simulink subsystem "Final_Project_PreAlign_20260605_152612"  (R2024a)
settings: Solver=VariableStepAuto  StartTime=0.0  StopTime=10.0  RelTol=1e-3
values from neighbouring files (symbols this model uses):
  D = hypot(Ep(:,1)-Tp(:,1)',Ep(:,2)-Tp(:,2)')    [pp_compare_stage.m]    (also in pp_diag_path.m; pp_t09_clear.m = hypot(Ep(:,1)-Tperim(:,1)', Ep(:,2)-Tperim(:,2)'); pp_tune2.m)
undefined symbols (not defined in the file or in its folder): waypoint_const
libraries: CarMaker4SL x83, simulink x2
(part 4 of 5)

== matlab function Final_Project_PreAlign_20260605_152612/Driving_Module_Ver.3_PSH/Subsystem/Controller ==
  data: ego_cross_track_err input; steer output; ego_head_err input; ego_max_curvature input; target_speed input; lead_dist input; lead_speed input; drive_state input; lane_settled input; submission_state input; ego_state input; accel output; front_dist_lock output; gear_pos output double
function [steer, accel, front_dist_lock, gear_pos] = controller(...
    ego_cross_track_err, ego_head_err, ego_max_curvature, target_speed, ...
    lead_dist, lead_speed, drive_state, lane_settled, submission_state, ego_state)
%#codegen

    % ============================================================
    % 기본 상수
    % ============================================================
    TS           = 0.01;
    STEER_LIM    = 0.58;
    MAX_SPEED    = 50.0;
    MODE_LCHG    = int32(1);
    MODE_PARK    = int32(2);
    KAPPA_EPS    = 1e-4;
    SPD_DEADBAND = 0.3;

    % ============================================================
    % Cmd 정의
    % 0 : 일반 주행
    % 1 : 주차장 진입
    % 2 : 톨게이트
    % ============================================================
    CMD_DRIVE = int32(0); %#ok<NASGU>
    CMD_PARK  = int32(1);
    CMD_TOLL  = int32(2);

    submission_i = int32(round(double(submission_state)));

    mandatory_follow = (submission_i == CMD_PARK) || (submission_i == CMD_TOLL);

    % ============================================================
    % Ego unpack
    % ============================================================
    ego_x = ego_state.Car_Fr1_tx;
    ego_y = ego_state.Car_Fr1_ty;
    ego_v = ego_state.Ego_V;

    if ego_v > 60.0
        ego_v = ego_v / 3.6;
    end

    if ego_v < 0.0
        ego_v = 0.0;
    end

    % ============================================================
    % Parking waypoints
    % ============================================================
    L4_X     = -46.856;  L4_Y     = 15.842;
    L5_END_X =  2.617;   L5_END_Y = -35.0;

    dist_l4     = sqrt((ego_x - L4_X)^2     + (ego_y - L4_Y)^2);
    dist_to_end = sqrt((ego_x - L5_END_X)^2 + (ego_y - L5_END_Y)^2);

    % ============================================================
    % 파라미터 정의: 일반 주행 / 주차 진입
    % ============================================================
    K_STANLEY_NRM  = 0.88;   K_STANLEY_PRK  = 0.45;
    KP_HEAD_NRM    = 0.90;   KP_HEAD_PRK    = 0.50;
    LOOK_FRONT_NRM = calcLookFront(ego_v);  LOOK_FRONT_PRK = 10.0;
    ALAT_NRM       = 3.50;   ALAT_PRK       = 1.50;
    ATOT_NRM       = 4.00;   ATOT_PRK       = 2.00;
    MCSPD_NRM      = 7.00;   MCSPD_PRK      = 1.00;
    VREF_A_NRM     = 50.0;   VREF_A_PRK     = 2.00;
    VREF_D_NRM     = 100.0;  VREF_D_PRK     = 5.00;
    JERK_U_NRM     = 50.0;   JERK_U_PRK     = 3.00;
    JERK_D_NRM     = 60.0;   JERK_D_PRK     = 5.00;
    AMAX_NRM       = 10.0;   AMAX_PRK       = 3.00;
    DMAX_NRM       = 10.0;   DMAX_PRK       = 5.00;

    FADE_FAR  = 50.0;
    FADE_NEAR = 20.0;

    if submission_i == CMD_PARK
        if dist_l4 >= FADE_FAR
            r = 0.0;
        elseif dist_l4 <= FADE_NEAR
            r = 1.0;
        else
            r = (FADE_FAR - dist_l4) / (FADE_FAR - FADE_NEAR);
        end
    else
        r = 0.0;
    end

    K_STANLEY       = K_STANLEY_NRM  + r * (K_STANLEY_PRK  - K_STANLEY_NRM);
    KP_HEAD         = KP_HEAD_NRM    + r * (KP_HEAD_PRK    - KP_HEAD_NRM);
    LOOK_FRONT      = LOOK_FRONT_NRM + r * (LOOK_FRONT_PRK - LOOK_FRONT_NRM);
    A_LAT_LIMIT     = ALAT_NRM       + r * (ALAT_PRK       - ALAT_NRM);
    A_TOTAL_LIMIT   = ATOT_NRM       + r * (ATOT_PRK       - ATOT_NRM);
    MIN_CURVE_SPEED = MCSPD_NRM      + r * (MCSPD_PRK      - MCSPD_NRM);
    V_REF_ACCEL     = VREF_A_NRM     + r * (VREF_A_PRK     - VREF_A_NRM);
    V_REF_DECEL     = VREF_D_NRM     + r * (VREF_D_PRK     - VREF_D_NRM);
    JERK_UP         = JERK_U_NRM     + r * (JERK_U_PRK     - JERK_U_NRM);
    JERK_DOWN       = JERK_D_NRM     + r * (JERK_D_PRK     - JERK_D_NRM);
    ACCEL_MAX_BASE  = AMAX_NRM       + r * (AMAX_PRK       - AMAX_NRM);
    DECEL_MAX_BASE  = DMAX_NRM       + r * (DMAX_PRK       - DMAX_NRM);

    % ============================================================
    % L4 통과 latch
    % ============================================================
    persistent l4_passed_p l4_pass_init_p

    if isempty(l4_pass_init_p)
        l4_passed_p    = false;
        l4_pass_init_p = true;
    end

    if submission_i ~= CMD_PARK
        l4_passed_p = false;
    end

    L4_PASS_DIST = 3.0;

    if submission_i == CMD_PARK && dist_l4 < L4_PASS_DIST
        l4_passed_p = true;
    end

    % ============================================================
    % 목표속도 결정
    % ============================================================
    if submission_i == CMD_PARK

        DECEL_DIST = 25.0;
        STOP_DIST  =  2.0;

        SPD_BEFORE_L4_FAR  = 12.3;
        SPD_BEFORE_L4_NEAR = 4.8;
        SPD_AFTER_L4       = 5.8;
        SPD_PARK_INSIDE    = 4.2;

        if drive_state == MODE_PARK

            if dist_to_end < STOP_DIST
                ts = 0.0;
            elseif dist_to_end < DECEL_DIST
                ts = SPD_PARK_INSIDE * (dist_to_end / DECEL_DIST);
            else
                ts = SPD_PARK_INSIDE;
            end

        elseif l4_passed_p

            ts = SPD_AFTER_L4;

        elseif dist_l4 > FADE_NEAR

            if dist_l4 >= FADE_FAR
                ts = SPD_BEFORE_L4_FAR;
            else
                ts = SPD_BEFORE_L4_FAR + ...
                     (SPD_BEFORE_L4_NEAR - SPD_BEFORE_L4_FAR) * r;
            end

        else

            ts = SPD_AFTER_L4;

        end

    else

        ts = target_speed;

        if ts > 20.0
            ts = ts / 3.6;
        end

    end

    if ts > MAX_SPEED
        ts = MAX_SPEED;
    end

    if ts < 0.0
        ts = 0.0;
    end

    % ============================================================
    % persistent
    % ============================================================
    persistent desired_v_p accel_p did_init

    if isempty(did_init)
        desired_v_p = ego_v;
        accel_p     = 0.0;
        did_init    = true;
    end

    % ============================================================
    % 1. Stanley 조향
    % ============================================================
    v_safe = ego_v;

    if v_safe < 1.0
        v_safe = 1.0;
    end

    steer = KP_HEAD * ego_head_err - atan2(K_STANLEY * ego_cross_track_err, v_safe);

    if steer > STEER_LIM
        steer = STEER_LIM;
    elseif steer < -STEER_LIM
        steer = -STEER_LIM;
    end

    % ============================================================
    % 1-1. 끝점 추가 좌회전 블렌드
    % ============================================================
    EXTRA_DIST = 5.0;
    EXTRA_RAD  = pi / 3.0;

    if submission_i == CMD_PARK && drive_state == MODE_PARK
        if dist_to_end < EXTRA_DIST && dist_to_end > 0.0
            blend = 1.0 - (dist_to_end / EXTRA_DIST);
            steer = steer + blend * EXTRA_RAD;

            if steer > EXTRA_RAD
                steer = EXTRA_RAD;
            elseif steer < -EXTRA_RAD
                steer = -EXTRA_RAD;
            end
        end
    end

    % ============================================================
    % 2. 곡률 기반 목표속도 제한
    % ============================================================
    desired_v_raw = ts;

    if ego_max_curvature > KAPPA_EPS

        v_curve = sqrt(A_LAT_LIMIT / ego_max_curvature);

        if v_curve < MIN_CURVE_SPEED
            v_curve = MIN_CURVE_SPEED;
        end

        if v_curve < desired_v_raw
            desired_v_raw = v_curve;
        end
    end

    % ============================================================
    % 3. ACC 앞차 감속
    % ============================================================
    acc_active = false;

    if mandatory_follow

        LOOK_FRONT_ACC = LOOK_FRONT;

        if LOOK_FRONT_ACC < 45.0
            LOOK_FRONT_ACC = 45.0;
        end

        if lead_dist < LOOK_FRONT_ACC
            acc_active = true;
        end

    else

        if drive_state ~= MODE_PARK

            if lead_dist < LOOK_FRONT

                time_gap = 2.0;
                ACC_GAIN = 0.5;

                safe_v = lead_speed + (lead_dist - time_gap * ego_v) * ACC_GAIN;

                if safe_v < desired_v_raw
                    desired_v_raw = safe_v;
                end
            end
        end
    end

    if desired_v_raw < 0.0
        desired_v_raw = 0.0;
    end

    % ============================================================
    % 4. 목표속도 변화율 제한
    % ============================================================
    dv = desired_v_raw - desired_v_p;

    max_dv_up = V_REF_ACCEL * TS;
    max_dv_dn = V_REF_DECEL * TS;

    if dv > max_dv_up
        desired_v_p = desired_v_p + max_dv_up;
    elseif dv < -max_dv_dn
        desired_v_p = desired_v_p - max_dv_dn;
    else
        desired_v_p = desired_v_raw;
    end

    desired_v = desired_v_p;

    if mandatory_follow && acc_active
        desired_v_p = ego_v;
        desired_v   = ego_v;
    end

    % ============================================================
    % 5. 가감속
    % ============================================================
    spd_err = desired_v - ego_v;

    if mandatory_follow && acc_active

        lead_v = lead_speed;

        if lead_v > 60.0
            lead_v = lead_v / 3.6;
        end

        if lead_v < 0.0
            lead_v = 0.0;
        end

        TIME_GAP_MAND     = 2.0;
        STOP_BUFFER       = 6.0;
        LOW_SPEED_MIN_GAP = 10.0;

        safe_gap = STOP_BUFFER + TIME_GAP_MAND * ego_v;

        if ego_v < 6.0
            if safe_gap < LOW_SPEED_MIN_GAP
                safe_gap = LOW_SPEED_MIN_GAP;
            end
        end

        gap_err   = lead_dist - safe_gap;
        closing_v = ego_v - lead_v;

        if closing_v < 0.0
            closing_v = 0.0;
        end

        GAP_CLOSE = -1.5;
        GAP_FAR   =  4.0;

        ACC_FOLLOW_ACCEL_MAX = 0.35;
        ACC_MATCH_ACCEL_MAX  = 0.20;
        ACC_FOLLOW_DECEL_MAX = 5.5;

        KP_FAR   = 0.05;
        KP_MATCH = 0.60;
        KP_CLOSE = 0.35;
        KD_CLOSE = 1.40;

        if gap_err > GAP_FAR

            accel_cmd = KP_FAR * (gap_err - GAP_FAR);

            if accel_cmd > ACC_FOLLOW_ACCEL_MAX
                accel_cmd = ACC_FOLLOW_ACCEL_MAX;
            end

            MAX_CATCHUP_V = 0.5;

            if ego_v > lead_v + MAX_CATCHUP_V
                accel_cmd = 0.0;
            end

        elseif gap_err < GAP_CLOSE

            accel_cmd = KP_CLOSE * gap_err - KD_CLOSE * closing_v;

            if accel_cmd < -ACC_FOLLOW_DECEL_MAX
                accel_cmd = -ACC_FOLLOW_DECEL_MAX;
            end

        else

            accel_cmd = KP_MATCH * (lead_v - ego_v);

            if accel_cmd > ACC_MATCH_ACCEL_MAX
                accel_cmd = ACC_MATCH_ACCEL_MAX;
            elseif accel_cmd < -ACC_FOLLOW_DECEL_MAX
                accel_cmd = -ACC_FOLLOW_DECEL_MAX;
            end
        end

        if lead_v < 0.3 && lead_dist < safe_gap + 5.0
            if accel_cmd > 0.0
                accel_cmd = 0.0;
            end
        end

        % 비상감속 조건 완화
        EMERGENCY_GAP = 5.0 + 0.5 * ego_v;

        if ego_v < 6.0
            EMERGENCY_GAP = 7.0 + 0.5 * ego_v;
        end

        if lead_dist < EMERGENCY_GAP && closing_v > 1.0
            accel_cmd = -ACC_FOLLOW_DECEL_MAX;
        end

    elseif submission_i == CMD_PARK

        KP_SPD = 2.0;
        accel_cmd = KP_SPD * spd_err;

        if accel_cmd > ACCEL_MAX_BASE
            accel_cmd = ACCEL_MAX_BASE;
        elseif accel_cmd < -DECEL_MAX_BASE
            accel_cmd = -DECEL_MAX_BASE;
        end

    else

        if spd_err > SPD_DEADBAND
            accel_cmd = ACCEL_MAX_BASE;
        elseif spd_err < -SPD_DEADBAND
            accel_cmd = -DECEL_MAX_BASE;
        else
            accel_cmd = 0.5 * spd_err;
        end
    end

    % ============================================================
    % 6. Friction circle 기반 가속 한계
    % ============================================================
    a_lat_now = ego_v * ego_v * ego_max_curvature;

    if a_lat_now >= A_TOTAL_LIMIT
        a_lon_avail = 0.5;
    else
        a_lon_avail = sqrt(A_TOTAL_LIMIT * A_TOTAL_LIMIT - a_lat_now * a_lat_now);

        if a_lon_avail < 0.5
            a_lon_avail = 0.5;
        end
    end

    accel_max = ACCEL_MAX_BASE;

    if a_lon_avail < accel_max
        accel_max = a_lon_avail;
    end

    if accel_cmd > accel_max
        accel_cmd = accel_max;
    end

    if accel_cmd < -DECEL_MAX_BASE
        accel_cmd = -DECEL_MAX_BASE;
    end

    % ============================================================
    % 7. Jerk 제한
    % ============================================================
    da = accel_cmd - accel_p;

    if mandatory_follow && acc_active

        FOLLOW_JERK_UP      = 0.8;
        FOLLOW_JERK_RELEASE = 4.0;
        FOLLOW_JERK_DOWN    = 80.0;

        if accel_p < 0.0
            max_da_up = FOLLOW_JERK_RELEASE * TS;
        else
            max_da_up = FOLLOW_JERK_UP * TS;
        end

        max_da_dn = FOLLOW_JERK_DOWN * TS;

    else

        max_da_up = JERK_UP   * TS;
        max_da_dn = JERK_DOWN * TS;
    end

    if da > max_da_up
        accel_p = accel_p + max_da_up;
    elseif da < -max_da_dn
        accel_p = accel_p - max_da_dn;
    else
        accel_p = accel_cmd;
    end

    accel = accel_p;

    % ============================================================
    % 8. front_dist_lock
    % ============================================================
    if drive_state == MODE_LCHG || lane_settled
        front_dist_lock = 0;
    else
        front_dist_lock = lead_dist;
    end

    % ============================================================
    % 9. Gear Position
    % ============================================================
    gear_pos = double(1);

end


function LOOK_FRONT = calcLookFront(v)
%#codegen

    v = abs(v);

    if v > 60.0
        v = v / 3.6;
    end

    V_HIGH = 80.0 / 3.6;

    if v < V_HIGH
        LOOK_FRONT = 25.0 + 1.0 * v;
    else
        LOOK_FRONT = 50.0 + 1.0 * V_HIGH + 30.0 * (v - V_HIGH);
    end

    if LOOK_FRONT > 120.0
        LOOK_FRONT = 120.0;
    end

end

== matlab function Final_Project_PreAlign_20260605_152612/Module_Selector/parking_entry_selector ==
  data: parking_map input; module_select output; parking_goal input; parking_start input; ego_global_pos input; waypoints input
function module_select = parking_entry_selector(parking_map, parking_goal, parking_start, ego_global_pos, waypoints) %#codegen
% Module_Selector 상태 (출력 module_select):
%   0 = Driving, 1 = Parking(도달 시 래치 고정), 2 = Tollgate(구간), 3 = 주차목표 도달(래치 고정)
%   톨게이트: (-94.9269,-159.103) 도달 -> 2,  (-172.724,-86.2036) 통과 -> 0
%   주차    : (-141.562,-17.5155) 도달 -> 1 로 래치
%   주차목표: (-2.92924, 9.6997) 도달 -> 3 으로 래치 (최우선)
%   ego_global_pos = [x; y] (Bus Selector+Mux)

persistent parking_latched tollgate_active goal_latched
if isempty(parking_latched)
    parking_latched = false;
end
if isempty(tollgate_active)
    tollgate_active = false;
end
if isempty(goal_latched)
    goal_latched = false;
end

TG_START = [-94.9269, -159.103];   % 톨게이트 시작
TG_END   = [-172.724,  -86.2036];  % 톨게이트 끝
PARK_REF = [-141.562,  -17.5155];  % 주차 진입
GOAL_REF = [1.81923,    -36.6415];  % 주차 목표 지점 (state 3)
R = 6.0;                           % 도달 인정 반경 [m] (자차가 ~5m 옆으로 지나가서 키움)
R_GOAL = 3.0;                      % 주차 목표 도달 반경 [m] (진입로 라인과 구분되도록 작게)

ex = ego_global_pos(1);
ey = ego_global_pos(2);

if hypot(ex - TG_START(1), ey - TG_START(2)) <= R
    tollgate_active = true;
end
if hypot(ex - TG_END(1), ey - TG_END(2)) <= R
    tollgate_active = false;
end

if hypot(ex - PARK_REF(1), ey - PARK_REF(2)) <= R
    parking_latched = true;
end

if hypot(ex - GOAL_REF(1), ey - GOAL_REF(2)) <= R_GOAL
    goal_latched = true;
end

if goal_latched
    module_select = 3.0;
elseif parking_latched
    module_select = 1.0;
elseif tollgate_active
    module_select = 2.0;
else
    module_select = 0.0;
end
end

== stateflow chart Final_Project_PreAlign_20260605_152612/FcnRouter_State ==
  (default) -> (junction 5)
  (junction 5) -> (junction 7) [order 1] : [isPark]{call_park;}
  (junction 5) -> (junction 8) [order 2] : [isPark == 0]{call_drive;}
  data: isPark input double
  events: tick input FUNCTION_CALL_EVENT; call_drive output FUNCTION_CALL_EVENT; call_park output FUNCTION_CALL_EVENT

== matlab function Final_Project_PreAlign_20260605_152612/Parking_system/MATLAB Function2 ==
  settings: sampleTime=0.05
  data: map_boundary input; mapMatrix output size=[200 200]; traffic_info input; traffic_size input
function mapMatrix = generate_map_(map_boundary, traffic_info, traffic_size)
%GENERATE_MAP_  Self-contained version of the "MATLAB Function1" block.
%   Source model : Models/Day4_5/Day4_5_Scenario_1.slx
%   Block path   : CarMaker/Subsystem/Day4 & 5/Scenario 1/MATLAB Function1
%
%   The block body only calls the pp_* helper; this file additionally
%   bundles every pp_*.m it transitively depends on as local functions,
%   so it runs standalone without dev/day4_5/pp_*.m on the MATLAB path.
%
%   Bundled dependencies (5): pp_generate_map, pp_cfg, pp_entrance_path, pp_grid2world, pp_world2grid
mapMatrix = pp_generate_map(map_boundary, traffic_info, traffic_size);
end

% ========================================================================
%  Local dependency functions (bundled verbatim from dev/day4_5/pp_*.m).
%  Do not edit here; edit the pp_*.m sources and re-bundle.
% ========================================================================

function mapMatrix = pp_generate_map(map_boundary, traffic_info, traffic_size) %#ok<INUSD>
%#codegen
% PP_GENERATE_MAP  Base occupancy grid for the parking area (M2 logic).
%   Output mapMatrix is n-by-n, indexed (iy, ix): 0 = free, 1 = occupied.
%
%   Drivable space = the parking-lot rectangle (cfg.lot) UNION the entrance-road
%   corridor (route5 centerline +- halfw, from pp_entrance_path), each inset by
%   cfg.edge_margin. Everything else inside cfg.bounds is OCCUPIED, so the planner
%   cannot cut across non-road area. Static parked cars are stamped afterwards by
%   pp_add_obstacle.
%
%   PERFORMANCE: the map is STATIC, so it is computed ONCE and cached in a
%   persistent (this block runs every sim step; the corridor distance-carve must
%   not run per-step). Codegen rule: the persistent is assigned inside the
%   `if isempty(...)` guard BEFORE it is read. Cache clears at sim start and by
%   `clear functions` after editing cfg / pp_entrance_path.
%
%   map_boundary / traffic_info / traffic_size are accepted only for MATLAB
%   Function block signature compatibility (intentionally unused here).
persistent BASE
if isempty(BASE)
    cfg = pp_cfg();
    n = cfg.n; b = cfg.bounds; em = cfg.edge_margin;
    M = ones(n, n);                                 % default OCCUPIED; carve drivable area free

    % --- carve the REAL drivable surface FREE (IPGRoad geometry, not a rectangle) -
    %   Driving lanes (type 0) + parking bay (type 13), reconstructed from the
    %   TestRun road links/lanes. surf rows = [x0 x1 y0 y1], ALREADY inset by the
    %   edge margin on OUTER paved walls only; internal seams (Vroad<->Hstrip and
    %   Hstrip<->Bay) are left flush so the vehicle can cross between them.
    %   Everything else inside cfg.bounds stays OCCUPIED (no cutting across void).
    %     Vroad : x~0 vertical driving road     world x[-2.5,2.5] y[-36.6,6]
    %     Hstrip: y~-36.6 driving strip (type0)  world x[0,47.6]   y[-39.1,-34.1]
    %     Bay   : type-13 parking bay (north)    world x[5.5,47.6] y[-34.1,-4.1]
    %     BayW  : narrow west sliver of the bay  world x[4,5.5]    y[-34.1,-30.1]
    surf = [ -2.3  2.3  -36.6    6.0 ;
              0.0 47.4  -38.9  -34.1 ;
              5.7 47.4  -34.1   -4.3 ;
              4.0  5.5  -34.1  -30.1 ];
    for r = 1:size(surf,1)
        [sx0, sy0] = pp_world2grid(surf(r,1), surf(r,3), b, n);
        [sx1, sy1] = pp_world2grid(surf(r,2), surf(r,4), b, n);
        for ix = min(sx0,sx1):max(sx0,sx1)
            for iy = min(sy0,sy1):max(sy0,sy1)
                M(iy, ix) = 0;
            end
        end
    end

    % --- occupied border ring (keeps the search bounded) ----------------------
    w = cfg.wall_cells;
    if w > 0
        M(1:w, :)     = 1;
        M(n-w+1:n, :) = 1;
        M(:, 1:w)     = 1;
        M(:, n-w+1:n) = 1;
    end

    BASE = M;
end
mapMatrix = BASE;
end

% ===== distance from point (px,py) to segment (ax,ay)-(bx,by) ==============
function d = seg_dist_(px, py, ax, ay, bx, by)
%#codegen
vx = bx-ax; vy = by-ay;
wx = px-ax; wy = py-ay;
vv = vx*vx + vy*vy;
if vv < 1e-9
    d = hypot(px-ax, py-ay); return;
end
t = (wx*vx + wy*vy) / vv;
if t < 0, t = 0; elseif t > 1, t = 1; end
qx = ax + t*vx; qy = ay + t*vy;
d = hypot(px-qx, py-qy);
end

function cfg = pp_cfg()
%#codegen
% PP_CFG  Configuration for the Day4/5 precise-parking controller (Kia_EV6).
%   Geometry from Data/Vehicle/Kia_EV6 (Vehicle.OuterSkin & wheel positions).
%
%   Pose convention (CarMaker): Car.Fr1 origin = REAR-BUMPER center on the road,
%   X forward, Y left, yaw = Car.Fr1.rz [rad]. Same convention for the mission
%   goal pose and every obstacle coordinate. Internal planning/tracking uses the
%   REAR AXLE, d_r ahead of Fr1:  rear_axle = Fr1 + d_r*[cos(yaw) sin(yaw)].
%
%   CODEGEN NOTE: build every struct field from LOCAL variables / literals only.
%   Never read a cfg field while still constructing cfg.

% --- local geometry constants (Kia_EV6) -----------------------------------
veh_L     = 4.68;
veh_W     = 1.88;
wheelbase = 2.90;
d_r       = 0.95;
delta_max = 30*pi/180;

% --- vehicle ---------------------------------------------------------------
cfg.veh_L       = veh_L;
cfg.veh_W       = veh_W;
cfg.veh_halfW   = veh_W/2;
cfg.wheelbase   = wheelbase;
cfg.track_f     = 1.624;                  % front track width [m] (wheels at y=+-0.812)
cfg.d_r         = d_r;
cfg.foot_ahead  = veh_L - d_r;            % rear-axle -> front bumper [m] = 3.73
cfg.foot_behind = d_r;                    % rear-axle -> rear bumper  [m] = 0.95
cfg.delta_max   = delta_max;
cfg.Rmin        = wheelbase / tan(delta_max);

% --- obstacle vehicle (IPG_CompanyCar_2018_Blue) ---------------------------
cfg.obs_L       = 4.47;
cfg.obs_W       = 1.97;
cfg.holdout     = 0;                     % pp_obstacles row kept FREE as the parking
                                          %   target (held-out car). 14 = T13. 0 = none.

% --- occupancy grid --------------------------------------------------------
cfg.n           = 200;                    % cells/side (occ_map [200 200]) -- keep 200: EML occ port is fixed
cfg.margin      = 0.40;                   % obstacle footprint safety inflation [m] (buffer for tracking error)
cfg.bounds      = [-5 48 -45.5 6];        % world planning rect [xmin xmax ymin ymax] = lot + NORTH entrance approach
                                          %   (res 53/200=0.265 x 51.5/200=0.258 m)
cfg.lot         = [2 48 -38 -3];          % drivable parking-lot rectangle (bottom raised -45.5->-38: real road ends ~ -37..-40, wall-crash fix)
cfg.edge_margin = 0.20;                    % safety margin inset from the drivable-region boundary (lot edges + corridor walls) [m]
cfg.wall_cells  = 1;                      % occupied border-ring thickness [cells]

% --- Hybrid A* planner -----------------------------------------------------
cfg.plan_res    = 0.5;                    % closed-set position resolution [m]
cfg.nxc         = 106;                    % closed-set X bins  ~ (bounds_x)/plan_res = 53/0.5
cfg.nyc         = 103;                    % closed-set Y bins  ~ (bounds_y)/plan_res = 51.5/0.5
cfg.nth         = 72;                     % heading bins (5 deg)
cfg.ds          = 0.6;                    % motion step (arc length) [m]
cfg.n_steer     = 5;                      % steering samples (odd, symmetric)
cfg.max_nodes   = 60000;                  % expansion / node cap
cfg.max_path    = 2000;                   % max stored path points
cfg.pos_tol     = 0.7;                    % planner goal position tol [m] (M9 refines)
cfg.yaw_tol     = 12*pi/180;              % planner goal heading tol [rad]
cfg.w_rev       = 2.0;                    % reverse cost multiplier
cfg.w_switch    = 2.0;                    % direction-change penalty [~m]
cfg.w_steer     = 0.3;                    % steering magnitude penalty
cfg.h_weight    = 1.2;                    % heuristic weight (>=1 speeds search)
cfg.rs_shot_dist = 15.0;                  % try RS one-shot to goal within this dist [m]
cfg.rs_heur_dist = 25.0;                  % use RS (vs Euclidean) heuristic within [m]

% --- M7 path tracking + longitudinal control -------------------------------
cfg.Ld          = 1.5;                    % (legacy) nominal lookahead [m]
cfg.Ld_min      = 0.5;                    % min lookahead (tight low-speed tracking) [m]
cfg.Ld_max      = 1.8;                    % max lookahead [m]
cfg.kld         = 1.2;                    % lookahead gain vs |speed| (Ld = Ld_min + kld*|v|)
cfg.v_fwd       = 1.0;                    % forward cruise speed [m/s] (faster approach)
cfg.v_rev       = 0.2;                    % reverse cruise speed [m/s] (known-good; speed-up revisited separately)
cfg.v_creep     = 0.10;                   % min creep speed while cruising [m/s]
cfg.v_stop      = 0.10;                   % treated as stopped [m/s]
cfg.kp_v        = 0.6;                    % longitudinal P gain (outer speed loop)
cfg.ax_max      = 0.6;                    % accel/brake command limit [m/s^2]
cfg.ax_min      = -1.5;                   % emergency decel/brake limit [m/s^2]
cfg.v_emax      = 1.2;                    % over-speed guard -> emergency brake [m/s]
cfg.v_obrake    = 0.40;                   % SAFETY-NET margin over target -> hard brake [m/s] (PI handles normal regulation)
cfg.ax_brake    = 1.5;                    % safety-net brake demand magnitude [m/s^2] (gear-dir: -ve = brake)
cfg.d_slow      = 5.0;                    % slow-down distance before cusp/goal [m] (weak brake -> decelerate early)
cfg.cusp_reach  = 0.30;                   % distance to register a cusp reached [m]
cfg.goal_reach  = 0.08;                   % path-end position tol [m]
cfg.max_rounds  = 4;                      % max RS corrective rounds in ALIGN (few shifts)

% --- M9 precise pose alignment (Astolfi pose regulation) -------------------
cfg.align_dist  = 3.0;                    % switch to alignment within this dist [m]
cfg.align_pos   = 0.08;                   % alignment done position tol [m]
cfg.align_yaw   = 2*pi/180;               % alignment done heading tol [rad]
cfg.v_align     = 0.3;                    % alignment creep speed [m/s]
cfg.v_align_min = 0.15;                   % min alignment creep speed [m/s]
cfg.kr          = 0.5;                    % Astolfi rho gain (approach)
cfg.ka          = 1.5;                    % Astolfi alpha gain (bearing)
cfg.kb          = -0.5;                   % Astolfi beta gain (final heading, <0)

% --- CarMaker gear selector enum (include/Vehicle.h) -----------------------
cfg.GEAR_P      = -9;
cfg.GEAR_R      = -1;
cfg.GEAR_N      = 0;
cfg.GEAR_D      = 1;
end

function [WP, nW, halfw] = pp_entrance_path()
%#codegen
% PP_ENTRANCE_PATH  Baked centerline of the lot WEST/NORTH entrance road.
%   WP is nW-by-2 [x y] in the Car.Fr1 world frame (rear-bumper convention),
%   halfw = drivable corridor half-width [m]. pp_generate_map carves cells
%   within halfw of this polyline FREE (the rest of the approach stays occupied),
%   replacing the old "whole west strip is free" rectangle.
%   Source: src_cm4sl/map_data/final/ -- route5 centerline (final_map_waypoint_
%   raw_data.mat), width from left/right lane edges (final_map_raw_data.mat,
%   full road ~5.3 m). Northern approach truncated at y<=3.5 m to keep n=200
%   grid resolution; extend WP + cfg.bounds(4) north if the real start is higher.
WP = [ ...
   -0.851     3.445; ...
   -0.804     2.068; ...
   -0.830     0.629; ...
   -0.906    -0.866; ...
   -1.008    -2.409; ...
   -1.113    -3.990; ...
   -1.205    -5.600; ...
   -1.277    -7.231; ...
   -1.328    -8.875; ...
   -1.362   -10.527; ...
   -1.384   -12.178; ...
   -1.393   -13.819; ...
   -1.392   -15.446; ...
   -1.387   -17.060; ...
   -1.383   -18.655; ...
   -1.382   -20.198; ...
   -1.384   -21.659; ...
   -1.387   -23.036; ...
   -1.387   -24.337; ...
   -1.379   -25.578; ...
   -1.356   -26.774; ...
   -1.310   -27.938; ...
   -1.229   -29.080; ...
   -1.100   -30.200; ...
   -0.907   -31.294; ...
   -0.636   -32.353; ...
   -0.275   -33.376; ...
    0.187   -34.363; ...
    0.760   -35.309; ...
    1.441   -36.210; ...
    1.819   -36.641; ...
];
nW = size(WP,1);
halfw = 2.5;   % ~ measured half road width (full ~5.3 m); fits the 1.88 m car
end

function [x, y] = pp_grid2world(ix, iy, b, n)
%#codegen
% PP_GRID2WORLD  1-based grid indices -> world coordinates of the CELL CENTER.
%   b = [xmin xmax ymin ymax], n = cells per side.
resx = (b(2) - b(1)) / n;
resy = (b(4) - b(3)) / n;
x = b(1) + (ix - 0.5) * resx;
y = b(3) + (iy - 0.5) * resy;
end

function [ix, iy] = pp_world2grid(x, y, b, n)
%#codegen
% PP_WORLD2GRID  World (x,y) -> 1-based grid indices (ix along X/col, iy along Y/row).
%   b = [xmin xmax ymin ymax], n = cells per side. Indices clamped to [1,n].
resx = (b(2) - b(1)) / n;
resy = (b(4) - b(3)) / n;
ix = floor((x - b(1)) / resx) + 1;
iy = floor((y - b(3)) / resy) + 1;
ix = min(max(ix, 1), n);
iy = min(max(iy, 1), n);
end

== matlab function Final_Project_PreAlign_20260605_152612/Parking_system/MATLAB Function3 ==
  settings: sampleTime=0.1
  data: map input size=[200 200]; y output size=[200 200]; traffic_info input; traffic_size input
function y = add_obstacle_(map, traffic_info, traffic_size)
%ADD_OBSTACLE_  Self-contained version of the "MATLAB Function2" block.
%   Source model : Models/Day4_5/Day4_5_Scenario_1.slx
%   Block path   : CarMaker/Subsystem/Day4 & 5/Scenario 1/MATLAB Function2
%
%   The block body only calls the pp_* helper; this file additionally
%   bundles every pp_*.m it transitively depends on as local functions,
%   so it runs standalone without dev/day4_5/pp_*.m on the MATLAB path.
%
%   Bundled dependencies (8): pp_add_obstacle, pp_cfg, pp_fill_rect, pp_grid2world, pp_obstacles, pp_pt_in_quad, pp_rect_corners, pp_world2grid
y = pp_add_obstacle(map, traffic_info, traffic_size);
end

% ========================================================================
%  Local dependency functions (bundled verbatim from dev/day4_5/pp_*.m).
%  Do not edit here; edit the pp_*.m sources and re-bundle.
% ========================================================================

function y = pp_add_obstacle(map, traffic_info, traffic_size) %#ok<INUSD>
%#codegen
% PP_ADD_OBSTACLE  Mark static parking obstacles onto the base map (M3 logic).
%   y = map with each obstacle footprint rasterized as occupied (1).
%
%   Obstacles are static & known, so they come from pp_obstacles() (rear-bumper
%   reference), inflated by cfg.margin on every side. The model's built-in
%   traffic reader (T01..T07) does NOT match the final lot's 21 cars, so
%   traffic_info / traffic_size are intentionally unused (kept for block
%   signature compatibility). Wire live traffic here only if the reader is
%   extended to all lot obstacles.
%
%   PERFORMANCE: the result is STATIC (cars never move; base map is the cached
%   constant from pp_generate_map), so it is computed ONCE and cached. Codegen
%   rule: the persistent is assigned inside the `if isempty(...)` guard BEFORE it
%   is read. Cache clears at sim start and by `clear functions`.
persistent FULL
if isempty(FULL)
    cfg = pp_cfg();
    n = cfg.n;
    b = cfg.bounds;
    yy = map;
    OBST = pp_obstacles();
    ahead  = cfg.obs_L + cfg.margin;
    behind = cfg.margin;
    halfw  = cfg.obs_W/2 + cfg.margin;
    for k = 1:size(OBST, 1)
        if k == cfg.holdout, continue; end          % keep the target slot free
        c = pp_rect_corners(OBST(k,1), OBST(k,2), OBST(k,3), ahead, behind, halfw);
        yy = pp_fill_rect(yy, c, b, n, 1);
    end
    FULL = yy;
end
y = FULL;
end

function cfg = pp_cfg()
%#codegen
% PP_CFG  Configuration for the Day4/5 precise-parking controller (Kia_EV6).
%   Geometry from Data/Vehicle/Kia_EV6 (Vehicle.OuterSkin & wheel positions).
%
%   Pose convention (CarMaker): Car.Fr1 origin = REAR-BUMPER center on the road,
%   X forward, Y left, yaw = Car.Fr1.rz [rad]. Same convention for the mission
%   goal pose and every obstacle coordinate. Internal planning/tracking uses the
%   REAR AXLE, d_r ahead of Fr1:  rear_axle = Fr1 + d_r*[cos(yaw) sin(yaw)].
%
%   CODEGEN NOTE: build every struct field from LOCAL variables / literals only.
%   Never read a cfg field while still constructing cfg.

% --- local geometry constants (Kia_EV6) -----------------------------------
veh_L     = 4.68;
veh_W     = 1.88;
wheelbase = 2.90;
d_r       = 0.95;
delta_max = 30*pi/180;

% --- vehicle ---------------------------------------------------------------
cfg.veh_L       = veh_L;
cfg.veh_W       = veh_W;
cfg.veh_halfW   = veh_W/2;
cfg.wheelbase   = wheelbase;
cfg.track_f     = 1.624;                  % front track width [m] (wheels at y=+-0.812)
cfg.d_r         = d_r;
cfg.foot_ahead  = veh_L - d_r;            % rear-axle -> front bumper [m] = 3.73
cfg.foot_behind = d_r;                    % rear-axle -> rear bumper  [m] = 0.95
cfg.delta_max   = delta_max;
cfg.Rmin        = wheelbase / tan(delta_max);

% --- obstacle vehicle (IPG_CompanyCar_2018_Blue) ---------------------------
cfg.obs_L       = 4.47;
cfg.obs_W       = 1.97;
cfg.holdout     = 0;                     % pp_obstacles row kept FREE as the parking
                                          %   target (held-out car). 14 = T13. 0 = none.

% --- occupancy grid --------------------------------------------------------
cfg.n           = 200;                    % cells/side (occ_map [200 200]) -- keep 200: EML occ port is fixed
cfg.margin      = 0.40;                   % obstacle footprint safety inflation [m] (buffer for tracking error)
cfg.bounds      = [-5 48 -45.5 6];        % world planning rect [xmin xmax ymin ymax] = lot + NORTH entrance approach
                                          %   (res 53/200=0.265 x 51.5/200=0.258 m)
cfg.lot         = [2 48 -38 -3];          % drivable parking-lot rectangle (bottom raised -45.5->-38: real road ends ~ -37..-40, wall-crash fix)
cfg.edge_margin = 0.20;                    % safety margin inset from the drivable-region boundary (lot edges + corridor walls) [m]
cfg.wall_cells  = 1;                      % occupied border-ring thickness [cells]

% --- Hybrid A* planner -----------------------------------------------------
cfg.plan_res    = 0.5;                    % closed-set position resolution [m]
cfg.nxc         = 106;                    % closed-set X bins  ~ (bounds_x)/plan_res = 53/0.5
cfg.nyc         = 103;                    % closed-set Y bins  ~ (bounds_y)/plan_res = 51.5/0.5
cfg.nth         = 72;                     % heading bins (5 deg)
cfg.ds          = 0.6;                    % motion step (arc length) [m]
cfg.n_steer     = 5;                      % steering samples (odd, symmetric)
cfg.max_nodes   = 60000;                  % expansion / node cap
cfg.max_path    = 2000;                   % max stored path points
cfg.pos_tol     = 0.7;                    % planner goal position tol [m] (M9 refines)
cfg.yaw_tol     = 12*pi/180;              % planner goal heading tol [rad]
cfg.w_rev       = 2.0;                    % reverse cost multiplier
cfg.w_switch    = 2.0;                    % direction-change penalty [~m]
cfg.w_steer     = 0.3;                    % steering magnitude penalty
cfg.h_weight    = 1.2;                    % heuristic weight (>=1 speeds search)
cfg.rs_shot_dist = 15.0;                  % try RS one-shot to goal within this dist [m]
cfg.rs_heur_dist = 25.0;                  % use RS (vs Euclidean) heuristic within [m]

% --- M7 path tracking + longitudinal control -------------------------------
cfg.Ld          = 1.5;                    % (legacy) nominal lookahead [m]
cfg.Ld_min      = 0.5;                    % min lookahead (tight low-speed tracking) [m]
cfg.Ld_max      = 1.8;                    % max lookahead [m]
cfg.kld         = 1.2;                    % lookahead gain vs |speed| (Ld = Ld_min + kld*|v|)
cfg.v_fwd       = 1.0;                    % forward cruise speed [m/s] (faster approach)
cfg.v_rev       = 0.2;                    % reverse cruise speed [m/s] (known-good; speed-up revisited separately)
cfg.v_creep     = 0.10;                   % min creep speed while cruising [m/s]
cfg.v_stop      = 0.10;                   % treated as stopped [m/s]
cfg.kp_v        = 0.6;                    % longitudinal P gain (outer speed loop)
cfg.ax_max      = 0.6;                    % accel/brake command limit [m/s^2]
cfg.ax_min      = -1.5;                   % emergency decel/brake limit [m/s^2]
cfg.v_emax      = 1.2;                    % over-speed guard -> emergency brake [m/s]
cfg.v_obrake    = 0.40;                   % SAFETY-NET margin over target -> hard brake [m/s] (PI handles normal regulation)
cfg.ax_brake    = 1.5;                    % safety-net brake demand magnitude [m/s^2] (gear-dir: -ve = brake)
cfg.d_slow      = 5.0;                    % slow-down distance before cusp/goal [m] (weak brake -> decelerate early)
cfg.cusp_reach  = 0.30;                   % distance to register a cusp reached [m]
cfg.goal_reach  = 0.08;                   % path-end position tol [m]
cfg.max_rounds  = 4;                      % max RS corrective rounds in ALIGN (few shifts)

% --- M9 precise pose alignment (Astolfi pose regulation) -------------------
cfg.align_dist  = 3.0;                    % switch to alignment within this dist [m]
cfg.align_pos   = 0.08;                   % alignment done position tol [m]
cfg.align_yaw   = 2*pi/180;               % alignment done heading tol [rad]
cfg.v_align     = 0.3;                    % alignment creep speed [m/s]
cfg.v_align_min = 0.15;                   % min alignment creep speed [m/s]
cfg.kr          = 0.5;                    % Astolfi rho gain (approach)
cfg.ka          = 1.5;                    % Astolfi alpha gain (bearing)
cfg.kb          = -0.5;                   % Astolfi beta gain (final heading, <0)

% --- CarMaker gear selector enum (include/Vehicle.h) -----------------------
cfg.GEAR_P      = -9;
cfg.GEAR_R      = -1;
cfg.GEAR_N      = 0;
cfg.GEAR_D      = 1;
end

function map = pp_fill_rect(map, c, b, n, val)
%#codegen
% PP_FILL_RECT  Rasterize a filled (possibly rotated) rectangle onto the grid.
%   c   : 4-by-2 world corners. b,n : grid definition. val : value to write.
%   Cells whose center falls inside the quad are set to val. map is n-by-n,
%   indexed map(iy, ix) (row = Y index, col = X index).
ixv = zeros(1, 4); iyv = zeros(1, 4);
for k = 1:4
    [ixv(k), iyv(k)] = pp_world2grid(c(k,1), c(k,2), b, n);
end
imin = max(min(ixv), 1); imax = min(max(ixv), n);
jmin = max(min(iyv), 1); jmax = min(max(iyv), n);
for ix = imin:imax
    for iy = jmin:jmax
        [cx, cy] = pp_grid2world(ix, iy, b, n);
        if pp_pt_in_quad(cx, cy, c)
            map(iy, ix) = val;
        end
    end
end
end

function [x, y] = pp_grid2world(ix, iy, b, n)
%#codegen
% PP_GRID2WORLD  1-based grid indices -> world coordinates of the CELL CENTER.
%   b = [xmin xmax ymin ymax], n = cells per side.
resx = (b(2) - b(1)) / n;
resy = (b(4) - b(3)) / n;
x = b(1) + (ix - 0.5) * resx;
y = b(3) + (iy - 0.5) * resy;
end

function OBST = pp_obstacles()
%#codegen
% PP_OBSTACLES  Static parking-lot obstacle table for the mission.
%   Returns K-by-3 array, each row [x y yaw] = obstacle REAR-BUMPER center [m]
%   and heading [rad] (same convention as ego Car.Fr1).
%
% Values below are the IVS_Final_Project CarMaker scenario lot (T00..T15,
%   IPG_CompanyCar_2018_Blue), taken from Data/TestRun/IVS_Final_Project StartPos.
%   Footprint (length cfg.obs_L forward, width cfg.obs_W) is applied in
%   pp_add_obstacle; do NOT pre-offset here.
H = pi/2;
OBST = [ ...
    7.3  -28.7  -H;   % T00
   12.8   -6.8  -H;   % T01
   21.3   -6.6  -H;   % T02
   30.0   -6.5  -H;   % T03
   41.7   -6.3  -H;   % T04
   31.0  -33.5   H;   % T05
    7.0  -21.8   H;   % T06
   18.6  -21.8   H;   % T07
   24.3  -21.9   H;   % T08
   14.0  -21.9   H;   % T09
   38.8  -21.8   H;   % T10
   41.8  -21.8   H;   % T11
   11.0  -28.8  -H;   % T12
   24.3  -28.9  -H;   % T13
   41.6  -28.9  -H;   % T14
   15.0  -33.5   H];  % T15
end

function tf = pp_pt_in_quad(px, py, c)
%#codegen
% PP_PT_IN_QUAD  True if point (px,py) lies inside the convex quad c (4-by-2).
%   Winding-agnostic: inside iff the point is on the same side of all 4 edges.
s = zeros(1, 4);
for k = 1:4
    k2 = mod(k, 4) + 1;
    ex = c(k2,1) - c(k,1);
    ey = c(k2,2) - c(k,2);
    s(k) = ex*(py - c(k,2)) - ey*(px - c(k,1));
end
tf = all(s >= -1e-9) || all(s <= 1e-9);
end

function c = pp_rect_corners(x, y, yaw, ahead, behind, halfw)
%#codegen
% PP_RECT_CORNERS  World corners (4-by-2) of an oriented rectangle.
%   Local frame: X forward, Y left. Rectangle spans X in [-behind, +ahead]
%   and Y in [-halfw, +halfw], placed at pose (x, y, yaw).
%   Corner order: front-left, front-right, rear-right, rear-left (clockwise).
co = cos(yaw); si = sin(yaw);
lx = [ahead,  ahead, -behind, -behind];
ly = [halfw, -halfw, -halfw,   halfw];
c = zeros(4, 2);
for k = 1:4
    c(k,1) = x + co*lx(k) - si*ly(k);
    c(k,2) = y + si*lx(k) + co*ly(k);
end
end

function [ix, iy] = pp_world2grid(x, y, b, n)
%#codegen
% PP_WORLD2GRID  World (x,y) -> 1-based grid indices (ix along X/col, iy along Y/row).
%   b = [xmin xmax ymin ymax], n = cells per side. Indices clamped to [1,n].
resx = (b(2) - b(1)) / n;
resy = (b(4) - b(3)) / n;
ix = floor((x - b(1)) / resx) + 1;
iy = floor((y - b(3)) / resy) + 1;
ix = min(max(ix, 1), n);
iy = min(max(iy, 1), n);
end

== matlab function Final_Project_PreAlign_20260605_152612/Driving_Module_Ver.3_PSH/Mission_Controller ==
  data: submission_state output; ego_state input; mission_cmd input; submission_cmd input; mission_state output
function [submission_state, mission_state] = Mission_Controller( ...
    ego_state, mission_cmd, submission_cmd)
%#codegen

    % ============================================================
    % Mission State 정의
    % 0 : Driving
    % 1 : Parking
    % ============================================================
    MISSION_DRIVING = int32(0);
    MISSION_PARKING = int32(1);

    % ============================================================
    % Submission State 정의
    % 0 : Default
    % 1 : Parking Entry
    % 2 : Tollgate
    % ============================================================
    SUB_DEFAULT  = int32(0);
    SUB_PARK_ENT = int32(1);
    SUB_TOLLGATE = int32(2); %#ok<NASGU>

    % ============================================================
    % 주차장 입구 좌표
    % ============================================================
    L5_END_X =  2.617;
    L5_END_Y = -36.038;

    ARRIVE_DIST  = 2.5;     % 도착 판단 반경 [m]
    ARRIVE_SPEED = 0.001;   % 정지 판단 속도 [m/s]

    % ============================================================
    % Ego unpack
    % ============================================================
    ego_x = ego_state.Car_Fr1_tx;
    ego_y = ego_state.Car_Fr1_ty;
    ego_v = ego_state.Ego_V;

    % ============================================================
    % persistent
    % ============================================================
    persistent mission_p submission_p did_init

    if isempty(did_init)
        mission_p    = MISSION_DRIVING;
        submission_p = SUB_DEFAULT;
        did_init     = true;
    end

    % ============================================================
    % 외부 cmd 반영
    % parking으로 전환된 이후에는 외부 cmd가 덮어쓰지 못하게 막음
    % ============================================================
    if mission_p ~= MISSION_PARKING
        mission_p    = int32(mission_cmd);
        submission_p = int32(submission_cmd);
    end
 
    % ============================================================
    % 주차장 입구 도착 판단
    % 조건: L5_END 반경 이내 + 속도 거의 0
    % ============================================================
    dx = ego_x - L5_END_X;
    dy = ego_y - L5_END_Y;
    dist_to_end = sqrt(dx*dx + dy*dy);

    if dist_to_end < ARRIVE_DIST && abs(ego_v) < ARRIVE_SPEED
        mission_p    = MISSION_PARKING;
        submission_p = SUB_PARK_ENT;
    end

    % ============================================================
    % 출력
    % ============================================================
    mission_state    = double(mission_p);
    submission_state = double(submission_p);

end
